simulink model "NlinCloopintcontrol"  (R2021a)
settings: Solver=VariableStepAuto  StartTime=0.0  StopTime=100  MaxStep=0.01  RelTol=1e-3
values from neighbouring files (symbols this model uses):
  g = 9.8    [Linearmodel.m]
  J = diag([2.7,3.3,5.4])    [Linearmodel.m]
  Jinv = J^-1    [Linearmodel.m]
  m = 0.254    [Linearmodel.m]
  windforce = [1;1;0]    [Linearmodel.m]
settings Model: Creator=Sirius  LastModifiedBy=Sirius

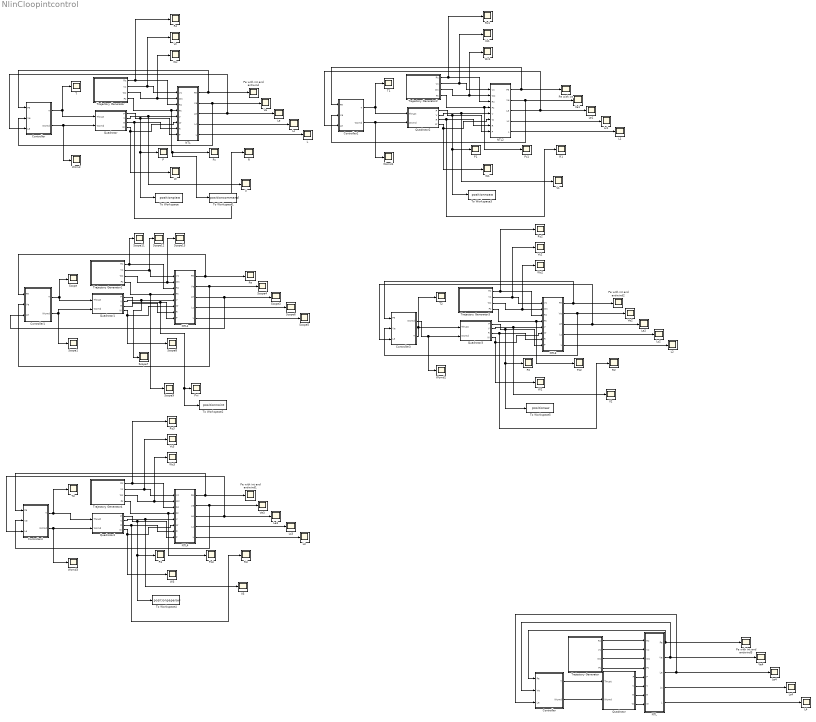
== system NlinCloopintcontrol ==
  Controller : Subsystem
  "Controller " : Subsystem
  Controller1 : MATLAB Function  TreatAsAtomicUnit=on
  Controller2 : Subsystem
  Controller3 : Subsystem
  Controller4 : Subsystem
  L{,1..4} (5 alike) : Scope
  Lc{,1..4} (5 alike) : Scope
  Le{,1..4} (5 alike) : Scope
  NTL : MATLAB Function  TreatAsAtomicUnit=on
  "NTL " : MATLAB Function  TreatAsAtomicUnit=on
  NTL1 : MATLAB Function  TreatAsAtomicUnit=on
  NTL2 : MATLAB Function  TreatAsAtomicUnit=on
  NTL3 : MATLAB Function  TreatAsAtomicUnit=on
  NTL4 : MATLAB Function  TreatAsAtomicUnit=on
  P{,1..3} (4 alike) : Scope
  Pc{,1..3} (4 alike) : Scope
  Pe : Scope
  Pe with int : Scope
  Pe with int and antiwind{,1..3} (4 alike) : Scope
  Pni : Scope
  Quadrotor : Subsystem
  "Quadrotor " : Subsystem
  Quadrotor1 : Subsystem
  Quadrotor2 : Subsystem
  Quadrotor3 : Subsystem
  Quadrotor4 : Subsystem
  R{,1..3} (4 alike) : Scope
  Rc{,1..3} (4 alike) : Scope
  Scope{,1,3..9,11..13} (12 alike) : Scope
  T{,1..3} (4 alike) : Scope
  To Workspace : ToWorkspace  VariableName=positionpiaw  SaveFormat=Timeseries  SampleTime=-1
  To Workspace1 : ToWorkspace  VariableName=positioncommand  SaveFormat=Timeseries  SampleTime=-1
  To Workspace2 : ToWorkspace  VariableName=positionnoint  SaveFormat=Timeseries  SampleTime=-1
  To Workspace3 : ToWorkspace  VariableName=positionnoaw  SaveFormat=Timeseries  SampleTime=-1
  To Workspace4 : ToWorkspace  VariableName=positionpaperaw  SaveFormat=Timeseries  SampleTime=-1
  To Workspace5 : ToWorkspace  VariableName=positionaw  SaveFormat=Timeseries  SampleTime=-1
  Trajectory Generator : Subsystem
  "Trajectory Generator " : Subsystem
  Trajectory Generator1 : Subsystem
  Trajectory Generator2 : Subsystem
  Trajectory Generator3 : Subsystem
  Trajectory Generator4 : Subsystem
  V{,1..3} (4 alike) : Scope
  Vc{,1..3} (4 alike) : Scope
  Ve{,1..4} (5 alike) : Scope
  W{,1..3} (4 alike) : Scope
  Wc{,1..3} (4 alike) : Scope
  Wcmd{,1..3} (4 alike) : Scope
  wires:
  Controller/1(T) -> Quadrotor/1(Thrust), T/1
  Trajectory Generator/3(Wc) -> Wc/1, NTL/2(Wc)
  Trajectory Generator/1(Rc) -> Rc/1, NTL/3(Rc)
  Trajectory Generator/4(Pc) -> To Workspace1/1, Pc/1, NTL/4(Pc)
  NTL/5(L) -> L/1
  NTL/4(Lc) -> Lc/1
  NTL/3(Le) -> Controller/3(Le), Le/1
  NTL/2(Ve) -> Controller/2(Ve), Ve/1
  NTL/1(Pe) -> Controller/1(Pe), Pe with int and antiwind/1
  Quadrotor/4(W) -> W/1, NTL/6(W)
  Quadrotor/1(P) -> P/1, To Workspace/1, NTL/8(P)
  Quadrotor/2(V) -> V/1, NTL/5(V)
  Quadrotor/3(R) -> R/1, NTL/7(R)
  Controller/2(Wcmd) -> Wcmd/1, Quadrotor/2(Wcmd)
  Trajectory Generator/2(Vc) -> Vc/1, NTL/1(Vc)
  Quadrotor1/4(W) -> Scope8/1, NTL1/6(W)
  Trajectory Generator1/4(Pc) -> Scope9/1, NTL1/4(Pc)
  Quadrotor1/1(P) -> To Workspace2/1, Pni/1, NTL1/8(P)
  Trajectory Generator1/1(Rc) -> Scope11/1, NTL1/3(Rc)
  Controller1/2(Wcmd) -> Quadrotor1/2(Wcmd), Scope1/1
  NTL1/1(Pe) -> Controller1/1(Pe), Pe/1
  Trajectory Generator1/3(Wc) -> Scope13/1, NTL1/2(Wc)
  Trajectory Generator1/2(Vc) -> Scope12/1, NTL1/1(Vc)
  NTL1/5(L) -> Scope5/1
  NTL1/2(Ve) -> Controller1/2(Ve), Scope4/1
  NTL1/3(Le) -> Controller1/3(Le), Scope3/1
  Controller1/1(T) -> Scope/1, Quadrotor1/1(Thrust)
  Quadrotor1/2(V) -> Scope7/1, NTL1/5(V)
  NTL1/4(Lc) -> Scope6/1
  Quadrotor1/3(R) -> NTL1/7(R)
  Quadrotor2/2(V) -> V1/1, NTL2/5(V)
  Controller2/2(Wcmd) -> Wcmd1/1, Quadrotor2/2(Wcmd)
  Controller2/1(T) -> Quadrotor2/1(Thrust), T1/1
  Trajectory Generator2/2(Vc) -> Vc1/1, NTL2/1(Vc)
  NTL2/1(Pe) -> Controller2/1(Pe), Pe with int/1
  Quadrotor2/3(R) -> R1/1, NTL2/7(R)
  Quadrotor2/1(P) -> P1/1, To Workspace3/1, NTL2/8(P)
  Trajectory Generator2/4(Pc) -> Pc1/1, NTL2/4(Pc)
  Trajectory Generator2/3(Wc) -> Wc1/1, NTL2/2(Wc)
  NTL2/4(Lc) -> Lc1/1
  NTL2/2(Ve) -> Controller2/2(Ve), Ve1/1
  NTL2/5(L) -> L1/1
  Quadrotor2/4(W) -> W1/1, NTL2/6(W)
  NTL2/3(Le) -> Controller2/3(Le), Le1/1
  Trajectory Generator2/1(Rc) -> Rc1/1, NTL2/3(Rc)
  NTL3/1(Pe) -> Controller3/1(Pe), Pe with int and antiwind2/1
  NTL3/3(Le) -> Controller3/3(Le), Le2/1
  Quadrotor3/1(P) -> P2/1, To Workspace5/1, NTL3/8(P)
  Trajectory Generator3/1(Rc) -> Rc2/1, NTL3/3(Rc)
  Quadrotor3/3(R) -> R2/1, NTL3/7(R)
  NTL3/2(Ve) -> Controller3/2(Ve), Ve2/1
  NTL3/5(L) -> L2/1
  Controller3/1(Wcmd) -> Wcmd2/1, Quadrotor3/2(Wcmd)
  Trajectory Generator3/3(Wc) -> Wc2/1, NTL3/2(Wc)
  Quadrotor3/2(V) -> V2/1, NTL3/5(V)
  Trajectory Generator3/2(Vc) -> Vc2/1, NTL3/1(Vc)
  Quadrotor3/4(W) -> W2/1, NTL3/6(W)
  NTL3/4(Lc) -> Lc2/1
  Trajectory Generator3/4(Pc) -> Pc2/1, NTL3/4(Pc)
  Controller3/2(T) -> Quadrotor3/1(Thrust), T2/1
  NTL4/1(Pe) -> Controller4/1(Pe), Pe with int and antiwind1/1
  NTL4/3(Le) -> Controller4/3(Le), Le3/1
  Quadrotor4/1(P) -> P3/1, To Workspace4/1, NTL4/8(P)
  Trajectory Generator4/1(Rc) -> Rc3/1, NTL4/3(Rc)
  Quadrotor4/3(R) -> R3/1, NTL4/7(R)
  NTL4/2(Ve) -> Controller4/2(Ve), Ve3/1
  NTL4/5(L) -> L3/1
  Trajectory Generator4/3(Wc) -> Wc3/1, NTL4/2(Wc)
  Quadrotor4/2(V) -> V3/1, NTL4/5(V)
  Trajectory Generator4/2(Vc) -> Vc3/1, NTL4/1(Vc)
  Quadrotor4/4(W) -> W3/1, NTL4/6(W)
  NTL4/4(Lc) -> Lc3/1
  Trajectory Generator4/4(Pc) -> Pc3/1, NTL4/4(Pc)
  Controller4/1(T) -> T3/1, Quadrotor4/1(Thrust)
  Controller4/2(Wcmd) -> Wcmd3/1, Quadrotor4/2(Wcmd)
  "Trajectory Generator "/1(Rc) -> "NTL "/1(Rc)
  "NTL "/5(L) -> L4/1
  "Quadrotor "/4(W) -> "NTL "/8(W)
  "Trajectory Generator "/2(Vc) -> "NTL "/2(Vc)
  "NTL "/2(Ve) -> Ve4/1, "Controller "/2(Ve)
  "Controller "/2(Wcmd) -> "Quadrotor "/2(Wcmd)
  "NTL "/1(Pe) -> Pe with int and antiwind3/1, "Controller "/1(Pe)
  "Quadrotor "/2(V) -> "NTL "/6(V)
  "NTL "/4(Lc) -> Lc4/1
  "Quadrotor "/3(R) -> "NTL "/7(R)
  "NTL "/3(Le) -> Le4/1, "Controller "/3(Le)
  "Trajectory Generator "/4(Pc) -> "NTL "/4(Pc)
  "Quadrotor "/1(P) -> "NTL "/5(P)
  "Controller "/1(T) -> "Quadrotor "/1(Thrust)
  "Trajectory Generator "/3(Wc) -> "NTL "/3(Wc)

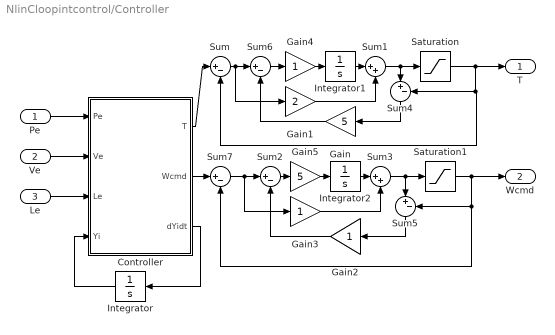
== system NlinCloopintcontrol/Controller ==
  Pe : Inport
  Ve : Inport  Port=2
  Le : Inport  Port=3
  Controller : MATLAB Function  TreatAsAtomicUnit=on
  Gain : Gain  Gain=5
  Gain1 : Gain  Gain=2
  Gain2 : Gain
  Gain3 : Gain
  Gain4 : Gain
  Gain5 : Gain  Gain=5
  Integrator : Integrator  InitialCondition=[0;0;0;0]
  Integrator1 : Integrator  InitialCondition=[0]
  Integrator2 : Integrator  InitialCondition=[0]
  Saturation : Saturate  UpperLimit=3  LowerLimit=-3
  Saturation1 : Saturate  UpperLimit=3  LowerLimit=-3
  Sum{,2,4..7} (6 alike) : Sum  Inputs=|+-
  Sum1 : Sum  Inputs=|++
  Sum3 : Sum  Inputs=|++
  T : Outport  VectorParamsAs1DForOutWhenUnconnected=off
  Wcmd : Outport  Port=2  VectorParamsAs1DForOutWhenUnconnected=off
  wires:
  Controller/3(dYidt) -> Integrator/1
  Integrator/1 -> Controller/4(Yi)
  Pe/1 -> Controller/1(Pe)
  Ve/1 -> Controller/2(Ve)
  Le/1 -> Controller/3(Le)
  Saturation/1 -> T/1, Sum/2, Sum4/2
  Controller/1(T) -> Sum/1
  Sum1/1 -> Saturation/1, Sum4/1
  Sum4/1 -> Gain/1
  Sum/1 -> Gain1/1, Sum6/1
  Gain4/1 -> Integrator1/1
  Sum2/1 -> Gain5/1
  Gain2/1 -> Sum2/2
  Sum3/1 -> Sum5/1, Saturation1/1
  Saturation1/1 -> Wcmd/1, Sum7/2, Sum5/2
  Gain5/1 -> Integrator2/1
  Sum5/1 -> Gain2/1
  Controller/2(Wcmd) -> Sum7/1
  Sum6/1 -> Gain4/1
  Gain/1 -> Sum6/2
  Sum7/1 -> Gain3/1, Sum2/1
  Integrator1/1 -> Sum1/1
  Gain1/1 -> Sum1/2
  Integrator2/1 -> Sum3/1
  Gain3/1 -> Sum3/2

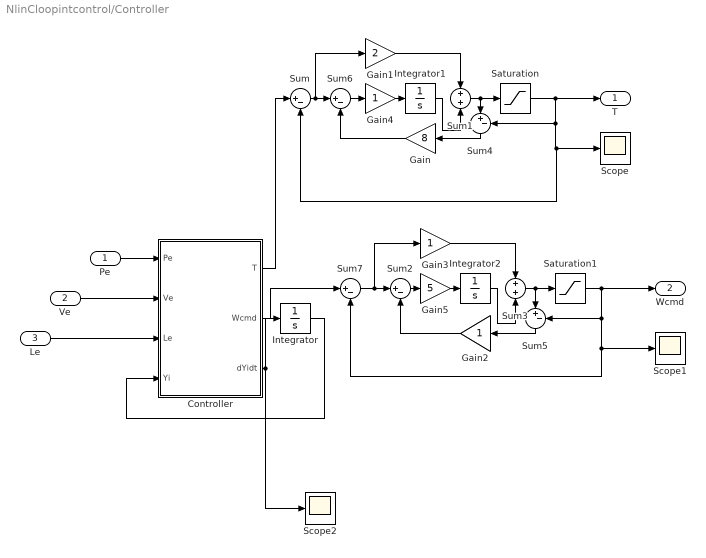
== system NlinCloopintcontrol/Controller  ==
  Pe : Inport
  Ve : Inport  Port=2
  Le : Inport  Port=3
  Controller : MATLAB Function  TreatAsAtomicUnit=on
  Gain : Gain  Gain=8
  Gain1 : Gain  Gain=2
  Gain2 : Gain
  Gain3 : Gain
  Gain4 : Gain
  Gain5 : Gain  Gain=5
  Integrator : Integrator  InitialCondition=[0;0;0;0]
  Integrator1 : Integrator  InitialCondition=[0]
  Integrator2 : Integrator  InitialCondition=[0]
  Saturation : Saturate  UpperLimit=3  LowerLimit=-3
  Saturation1 : Saturate  UpperLimit=3  LowerLimit=-3
  Scope : Scope
  Scope1 : Scope
  Scope2 : Scope
  Sum{,2,4..7} (6 alike) : Sum  Inputs=|+-
  Sum1 : Sum
  Sum3 : Sum
  T : Outport  VectorParamsAs1DForOutWhenUnconnected=off
  Wcmd : Outport  Port=2  VectorParamsAs1DForOutWhenUnconnected=off
  wires:
  Controller/3(dYidt) -> Integrator/1, Scope2/1
  Integrator/1 -> Controller/4(Yi)
  Pe/1 -> Controller/1(Pe)
  Ve/1 -> Controller/2(Ve)
  Le/1 -> Controller/3(Le)
  Saturation/1 -> T/1, Sum/2, Scope/1, Sum4/2
  Controller/1(T) -> Sum/1
  Gain1/1 -> Sum1/1
  Sum1/1 -> Saturation/1, Sum4/1
  Integrator1/1 -> Sum1/2
  Sum4/1 -> Gain/1
  Sum/1 -> Gain1/1, Sum6/1
  Gain4/1 -> Integrator1/1
  Sum2/1 -> Gain5/1
  Gain3/1 -> Sum3/1
  Gain2/1 -> Sum2/2
  Sum3/1 -> Sum5/1, Saturation1/1
  Integrator2/1 -> Sum3/2
  Saturation1/1 -> Wcmd/1, Sum7/2, Scope1/1, Sum5/2
  Gain5/1 -> Integrator2/1
  Sum5/1 -> Gain2/1
  Controller/2(Wcmd) -> Sum7/1
  Sum6/1 -> Gain4/1
  Gain/1 -> Sum6/2
  Sum7/1 -> Gain3/1, Sum2/1

== system NlinCloopintcontrol/Controller2 ==
  Pe : Inport
  Ve : Inport  Port=2
  Le : Inport  Port=3
  Controller : MATLAB Function  TreatAsAtomicUnit=on
  Integrator : Integrator  InitialCondition=[0;0;0;0]
  Scope : Scope
  Scope1 : Scope
  To Workspace : ToWorkspace  VariableName=xnoaw  SaveFormat=Timeseries  SampleTime=-1
  To Workspace1 : ToWorkspace  VariableName=unoaw  SaveFormat=Timeseries  SampleTime=-1
  T : Outport  VectorParamsAs1DForOutWhenUnconnected=off
  Wcmd : Outport  Port=2  VectorParamsAs1DForOutWhenUnconnected=off
  wires:
  Controller/3(dYidt) -> Integrator/1
  Integrator/1 -> Controller/4(Yi)
  Pe/1 -> Controller/1(Pe)
  Ve/1 -> Controller/2(Ve)
  Le/1 -> Controller/3(Le)
  Controller/4(x) -> To Workspace/1
  Controller/5(u) -> To Workspace1/1
  Controller/1(T) -> Scope/1, T/1
  Controller/2(Wcmd) -> Scope1/1, Wcmd/1

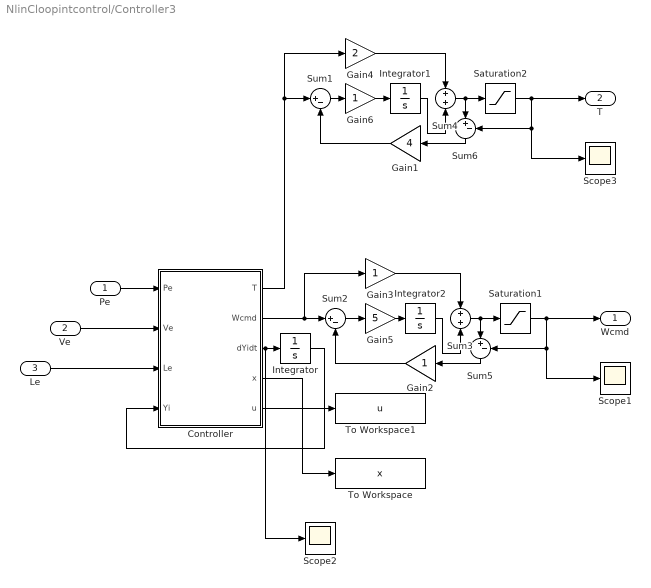
== system NlinCloopintcontrol/Controller3 ==
  Pe : Inport
  Ve : Inport  Port=2
  Le : Inport  Port=3
  Controller : MATLAB Function  TreatAsAtomicUnit=on
  Gain1 : Gain  Gain=4
  Gain2 : Gain
  Gain3 : Gain
  Gain4 : Gain  Gain=2
  Gain5 : Gain  Gain=5
  Gain6 : Gain
  Integrator : Integrator  InitialCondition=[0;0;0;0]
  Integrator1 : Integrator  InitialCondition=[0]
  Integrator2 : Integrator  InitialCondition=[0]
  Saturation1 : Saturate  UpperLimit=3  LowerLimit=-3
  Saturation2 : Saturate  UpperLimit=3  LowerLimit=-3
  Scope1 : Scope
  Scope2 : Scope
  Scope3 : Scope
  Sum{1..2,5..6} (4 alike) : Sum  Inputs=|+-
  Sum3 : Sum
  Sum4 : Sum
  To Workspace : ToWorkspace  VariableName=x  SaveFormat=Timeseries  SampleTime=-1
  To Workspace1 : ToWorkspace  VariableName=u  SaveFormat=Timeseries  SampleTime=-1
  Wcmd : Outport  VectorParamsAs1DForOutWhenUnconnected=off
  T : Outport  Port=2  VectorParamsAs1DForOutWhenUnconnected=off
  wires:
  Controller/3(dYidt) -> Scope2/1, Integrator/1
  Integrator/1 -> Controller/4(Yi)
  Pe/1 -> Controller/1(Pe)
  Ve/1 -> Controller/2(Ve)
  Le/1 -> Controller/3(Le)
  Controller/4(x) -> To Workspace/1
  Controller/5(u) -> To Workspace1/1
  Controller/1(T) -> Gain4/1, Sum1/1
  Sum2/1 -> Gain5/1
  Gain3/1 -> Sum3/1
  Gain2/1 -> Sum2/2
  Sum3/1 -> Sum5/1, Saturation1/1
  Integrator2/1 -> Sum3/2
  Saturation1/1 -> Wcmd/1, Scope1/1, Sum5/2
  Gain5/1 -> Integrator2/1
  Sum5/1 -> Gain2/1
  Controller/2(Wcmd) -> Gain3/1, Sum2/1
  Integrator1/1 -> Sum4/2
  Gain1/1 -> Sum1/2
  Gain4/1 -> Sum4/1
  Sum4/1 -> Sum6/1, Saturation2/1
  Saturation2/1 -> T/1, Scope3/1, Sum6/2
  Gain6/1 -> Integrator1/1
  Sum6/1 -> Gain1/1
  Sum1/1 -> Gain6/1

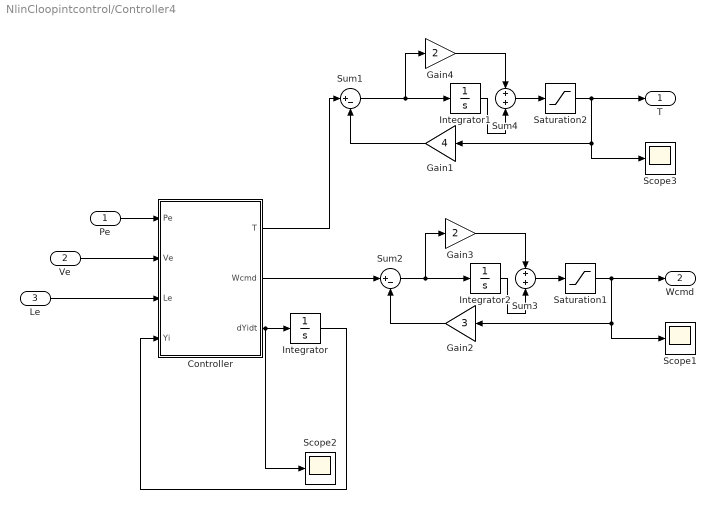
== system NlinCloopintcontrol/Controller4 ==
  Pe : Inport
  Ve : Inport  Port=2
  Le : Inport  Port=3
  Controller : MATLAB Function  TreatAsAtomicUnit=on
  Gain1 : Gain  Gain=4
  Gain2 : Gain  Gain=3
  Gain3 : Gain  Gain=2
  Gain4 : Gain  Gain=2
  Integrator : Integrator  InitialCondition=[0;0;0;0]
  Integrator1 : Integrator  InitialCondition=[0]
  Integrator2 : Integrator  InitialCondition=[0]
  Saturation1 : Saturate  UpperLimit=3  LowerLimit=-3
  Saturation2 : Saturate  UpperLimit=3  LowerLimit=-3
  Scope1 : Scope
  Scope2 : Scope
  Scope3 : Scope
  Sum1 : Sum  Inputs=|+-
  Sum2 : Sum  Inputs=|+-
  Sum3 : Sum
  Sum4 : Sum
  T : Outport  VectorParamsAs1DForOutWhenUnconnected=off
  Wcmd : Outport  Port=2  VectorParamsAs1DForOutWhenUnconnected=off
  wires:
  Controller/3(dYidt) -> Scope2/1, Integrator/1
  Pe/1 -> Controller/1(Pe)
  Ve/1 -> Controller/2(Ve)
  Le/1 -> Controller/3(Le)
  Controller/1(T) -> Sum1/1
  Controller/2(Wcmd) -> Sum2/1
  Sum4/1 -> Saturation2/1
  Integrator1/1 -> Sum4/2
  Gain4/1 -> Sum4/1
  Saturation2/1 -> T/1, Gain1/1, Scope3/1
  Sum1/1 -> Gain4/1, Integrator1/1
  Gain1/1 -> Sum1/2
  Integrator/1 -> Controller/4(Yi)
  Sum3/1 -> Saturation1/1
  Integrator2/1 -> Sum3/2
  Gain3/1 -> Sum3/1
  Saturation1/1 -> Wcmd/1, Gain2/1, Scope1/1
  Sum2/1 -> Gain3/1, Integrator2/1
  Gain2/1 -> Sum2/2

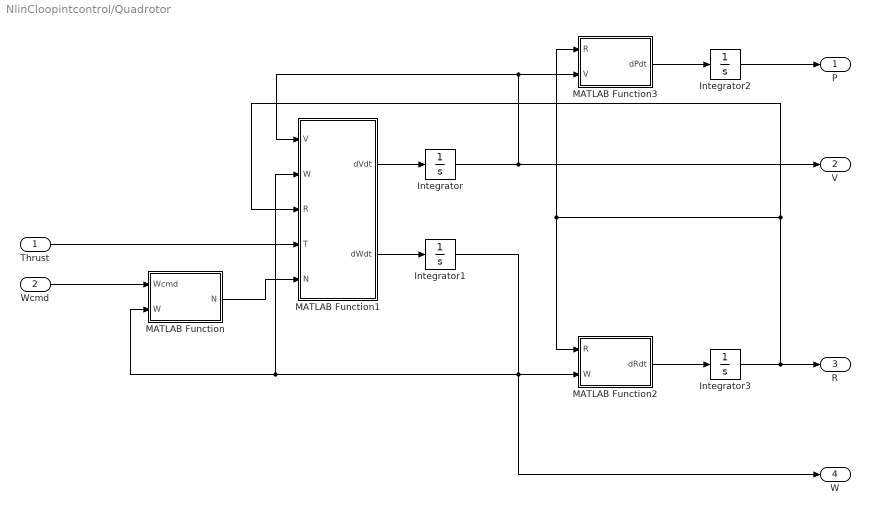
== system NlinCloopintcontrol/Quadrotor ==
  Thrust : Inport
  Wcmd : Inport  Port=2
  Integrator : Integrator  InitialCondition=[0;0;0]
  Integrator1 : Integrator  InitialCondition=[0;0;0]
  Integrator2 : Integrator  InitialCondition=[0;1;0]
  Integrator3 : Integrator  InitialCondition=eye(3)
  MATLAB Function : MATLAB Function  TreatAsAtomicUnit=on
  MATLAB Function1 : MATLAB Function  TreatAsAtomicUnit=on
  MATLAB Function2 : MATLAB Function  TreatAsAtomicUnit=on
  MATLAB Function3 : MATLAB Function  TreatAsAtomicUnit=on
  P : Outport
  V : Outport  Port=2
  R : Outport  Port=3
  W : Outport  Port=4
  wires:
  MATLAB Function2/1(dRdt) -> Integrator3/1
  Wcmd/1 -> MATLAB Function/1(Wcmd)
  MATLAB Function1/1(dVdt) -> Integrator/1
  Thrust/1 -> MATLAB Function1/4(T)
  MATLAB Function1/2(dWdt) -> Integrator1/1
  MATLAB Function/1(N) -> MATLAB Function1/5(N)
  MATLAB Function3/1(dPdt) -> Integrator2/1
  Integrator/1 -> V/1, MATLAB Function1/1(V), MATLAB Function3/2(V)
  Integrator3/1 -> MATLAB Function1/3(R), MATLAB Function3/1(R), MATLAB Function2/1(R), R/1
  Integrator1/1 -> MATLAB Function1/2(W), MATLAB Function/2(W), W/1, MATLAB Function2/2(W)
  Integrator2/1 -> P/1

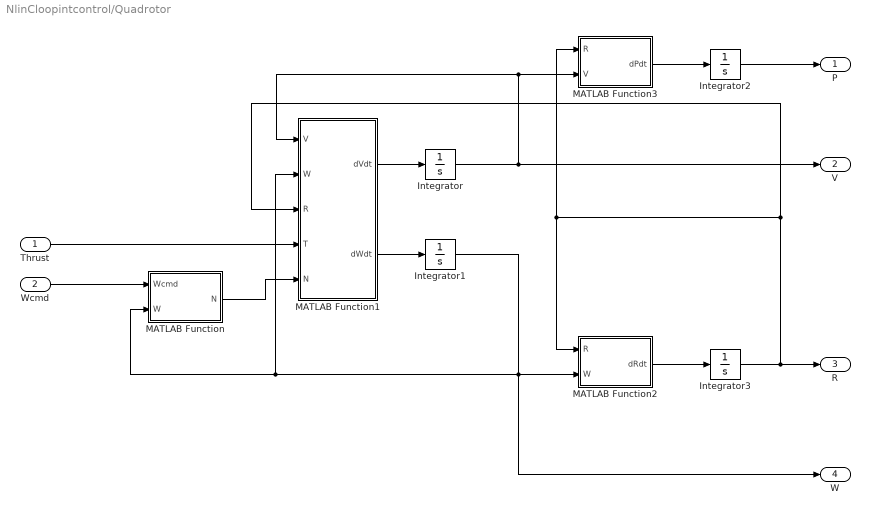
== system NlinCloopintcontrol/Quadrotor  ==
  Thrust : Inport
  Wcmd : Inport  Port=2
  Integrator : Integrator  InitialCondition=[0;0;0]
  Integrator1 : Integrator  InitialCondition=[0;0;0]
  Integrator2 : Integrator  InitialCondition=[0;1;0]
  Integrator3 : Integrator  InitialCondition=eye(3)
  MATLAB Function : MATLAB Function  TreatAsAtomicUnit=on
  MATLAB Function1 : MATLAB Function  TreatAsAtomicUnit=on
  MATLAB Function2 : MATLAB Function  TreatAsAtomicUnit=on
  MATLAB Function3 : MATLAB Function  TreatAsAtomicUnit=on
  P : Outport
  V : Outport  Port=2
  R : Outport  Port=3
  W : Outport  Port=4
  wires:
  MATLAB Function2/1(dRdt) -> Integrator3/1
  Wcmd/1 -> MATLAB Function/1(Wcmd)
  MATLAB Function1/1(dVdt) -> Integrator/1
  Thrust/1 -> MATLAB Function1/4(T)
  MATLAB Function1/2(dWdt) -> Integrator1/1
  MATLAB Function/1(N) -> MATLAB Function1/5(N)
  MATLAB Function3/1(dPdt) -> Integrator2/1
  Integrator/1 -> V/1, MATLAB Function1/1(V), MATLAB Function3/2(V)
  Integrator3/1 -> MATLAB Function1/3(R), MATLAB Function3/1(R), MATLAB Function2/1(R), R/1
  Integrator1/1 -> MATLAB Function1/2(W), MATLAB Function/2(W), W/1, MATLAB Function2/2(W)
  Integrator2/1 -> P/1

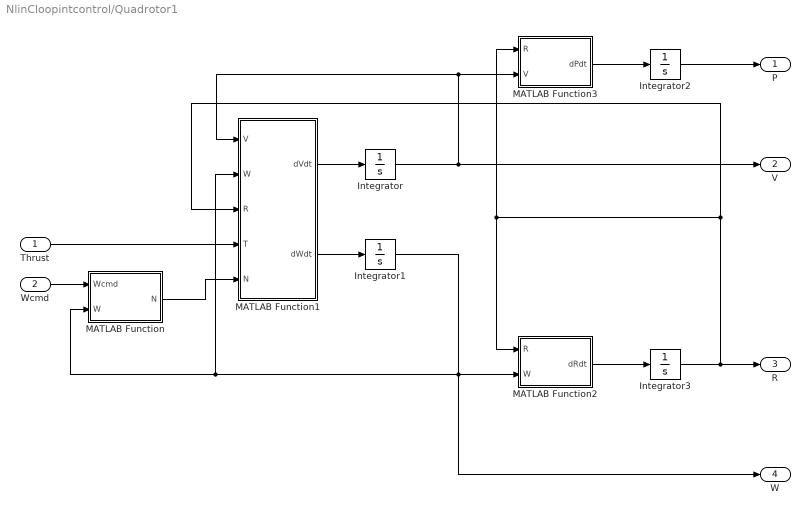
== system NlinCloopintcontrol/Quadrotor1 ==
  Thrust : Inport
  Wcmd : Inport  Port=2
  Integrator : Integrator  InitialCondition=[0;0;0]
  Integrator1 : Integrator  InitialCondition=[0;0;0]
  Integrator2 : Integrator  InitialCondition=[0;1;0]
  Integrator3 : Integrator  InitialCondition=eye(3)
  MATLAB Function : MATLAB Function  TreatAsAtomicUnit=on
  MATLAB Function1 : MATLAB Function  TreatAsAtomicUnit=on
  MATLAB Function2 : MATLAB Function  TreatAsAtomicUnit=on
  MATLAB Function3 : MATLAB Function  TreatAsAtomicUnit=on
  P : Outport
  V : Outport  Port=2
  R : Outport  Port=3
  W : Outport  Port=4
  wires:
  MATLAB Function2/1(dRdt) -> Integrator3/1
  Wcmd/1 -> MATLAB Function/1(Wcmd)
  MATLAB Function1/1(dVdt) -> Integrator/1
  Thrust/1 -> MATLAB Function1/4(T)
  MATLAB Function1/2(dWdt) -> Integrator1/1
  MATLAB Function/1(N) -> MATLAB Function1/5(N)
  MATLAB Function3/1(dPdt) -> Integrator2/1
  Integrator/1 -> V/1, MATLAB Function1/1(V), MATLAB Function3/2(V)
  Integrator3/1 -> MATLAB Function1/3(R), MATLAB Function3/1(R), MATLAB Function2/1(R), R/1
  Integrator1/1 -> MATLAB Function1/2(W), MATLAB Function/2(W), W/1, MATLAB Function2/2(W)
  Integrator2/1 -> P/1

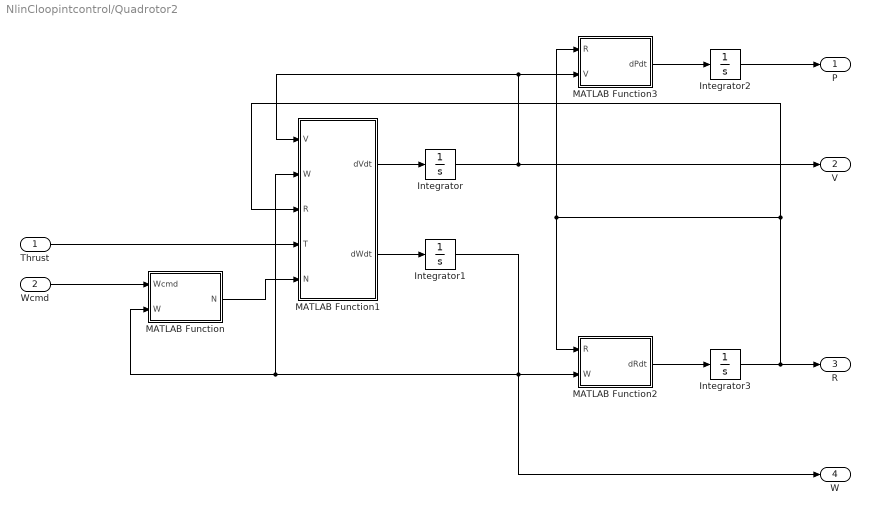
== system NlinCloopintcontrol/Quadrotor2 ==
  Thrust : Inport
  Wcmd : Inport  Port=2
  Integrator : Integrator  InitialCondition=[0;0;0]
  Integrator1 : Integrator  InitialCondition=[0;0;0]
  Integrator2 : Integrator  InitialCondition=[0;1;0]
  Integrator3 : Integrator  InitialCondition=eye(3)
  MATLAB Function : MATLAB Function  TreatAsAtomicUnit=on
  MATLAB Function1 : MATLAB Function  TreatAsAtomicUnit=on
  MATLAB Function2 : MATLAB Function  TreatAsAtomicUnit=on
  MATLAB Function3 : MATLAB Function  TreatAsAtomicUnit=on
  P : Outport
  V : Outport  Port=2
  R : Outport  Port=3
  W : Outport  Port=4
  wires:
  MATLAB Function2/1(dRdt) -> Integrator3/1
  Wcmd/1 -> MATLAB Function/1(Wcmd)
  MATLAB Function1/1(dVdt) -> Integrator/1
  Thrust/1 -> MATLAB Function1/4(T)
  MATLAB Function1/2(dWdt) -> Integrator1/1
  MATLAB Function/1(N) -> MATLAB Function1/5(N)
  MATLAB Function3/1(dPdt) -> Integrator2/1
  Integrator/1 -> V/1, MATLAB Function1/1(V), MATLAB Function3/2(V)
  Integrator3/1 -> MATLAB Function1/3(R), MATLAB Function3/1(R), MATLAB Function2/1(R), R/1
  Integrator1/1 -> MATLAB Function1/2(W), MATLAB Function/2(W), W/1, MATLAB Function2/2(W)
  Integrator2/1 -> P/1

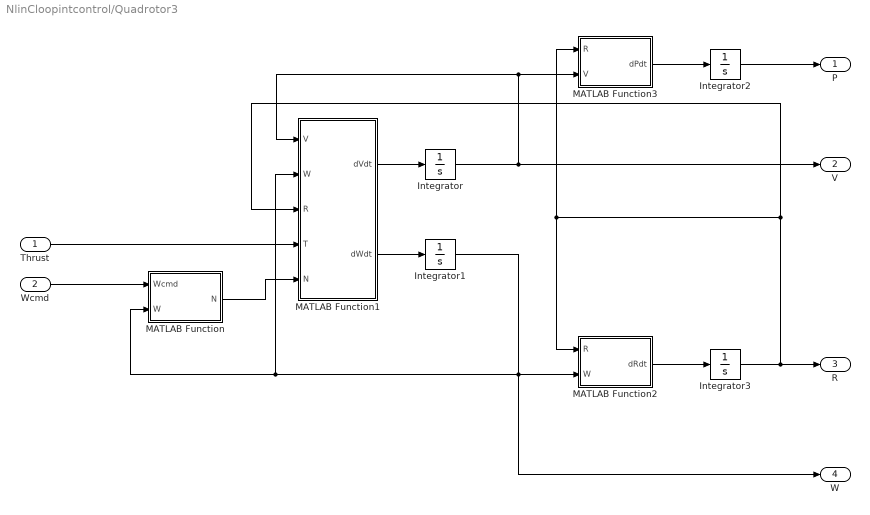
== system NlinCloopintcontrol/Quadrotor3 ==
  Thrust : Inport
  Wcmd : Inport  Port=2
  Integrator : Integrator  InitialCondition=[0;0;0]
  Integrator1 : Integrator  InitialCondition=[0;0;0]
  Integrator2 : Integrator  InitialCondition=[0;1;0]
  Integrator3 : Integrator  InitialCondition=eye(3)
  MATLAB Function : MATLAB Function  TreatAsAtomicUnit=on
  MATLAB Function1 : MATLAB Function  TreatAsAtomicUnit=on
  MATLAB Function2 : MATLAB Function  TreatAsAtomicUnit=on
  MATLAB Function3 : MATLAB Function  TreatAsAtomicUnit=on
  P : Outport
  V : Outport  Port=2
  R : Outport  Port=3
  W : Outport  Port=4
  wires:
  MATLAB Function2/1(dRdt) -> Integrator3/1
  Wcmd/1 -> MATLAB Function/1(Wcmd)
  MATLAB Function1/1(dVdt) -> Integrator/1
  Thrust/1 -> MATLAB Function1/4(T)
  MATLAB Function1/2(dWdt) -> Integrator1/1
  MATLAB Function/1(N) -> MATLAB Function1/5(N)
  MATLAB Function3/1(dPdt) -> Integrator2/1
  Integrator/1 -> V/1, MATLAB Function1/1(V), MATLAB Function3/2(V)
  Integrator3/1 -> MATLAB Function1/3(R), MATLAB Function3/1(R), MATLAB Function2/1(R), R/1
  Integrator1/1 -> MATLAB Function1/2(W), MATLAB Function/2(W), W/1, MATLAB Function2/2(W)
  Integrator2/1 -> P/1

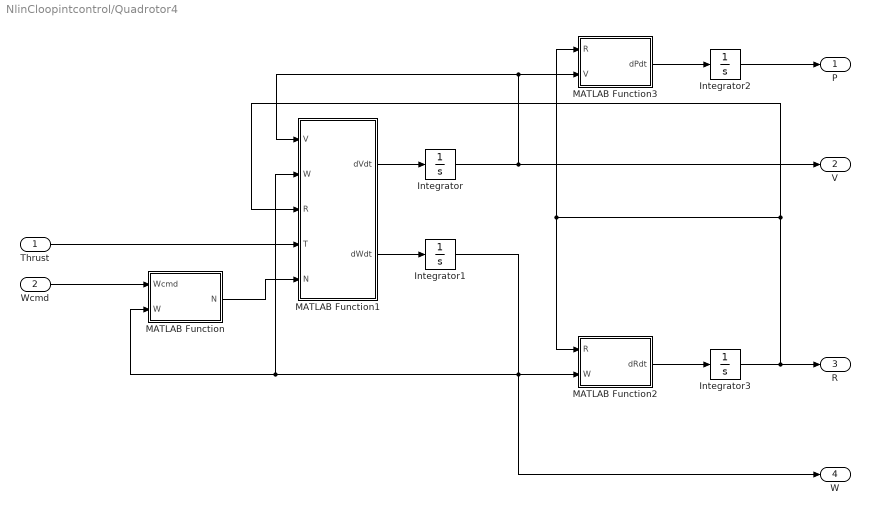
== system NlinCloopintcontrol/Quadrotor4 ==
  Thrust : Inport
  Wcmd : Inport  Port=2
  Integrator : Integrator  InitialCondition=[0;0;0]
  Integrator1 : Integrator  InitialCondition=[0;0;0]
  Integrator2 : Integrator  InitialCondition=[0;1;0]
  Integrator3 : Integrator  InitialCondition=eye(3)
  MATLAB Function : MATLAB Function  TreatAsAtomicUnit=on
  MATLAB Function1 : MATLAB Function  TreatAsAtomicUnit=on
  MATLAB Function2 : MATLAB Function  TreatAsAtomicUnit=on
  MATLAB Function3 : MATLAB Function  TreatAsAtomicUnit=on
  P : Outport
  V : Outport  Port=2
  R : Outport  Port=3
  W : Outport  Port=4
  wires:
  MATLAB Function2/1(dRdt) -> Integrator3/1
  Wcmd/1 -> MATLAB Function/1(Wcmd)
  MATLAB Function1/1(dVdt) -> Integrator/1
  Thrust/1 -> MATLAB Function1/4(T)
  MATLAB Function1/2(dWdt) -> Integrator1/1
  MATLAB Function/1(N) -> MATLAB Function1/5(N)
  MATLAB Function3/1(dPdt) -> Integrator2/1
  Integrator/1 -> V/1, MATLAB Function1/1(V), MATLAB Function3/2(V)
  Integrator3/1 -> MATLAB Function1/3(R), MATLAB Function3/1(R), MATLAB Function2/1(R), R/1
  Integrator1/1 -> MATLAB Function1/2(W), MATLAB Function/2(W), W/1, MATLAB Function2/2(W)
  Integrator2/1 -> P/1

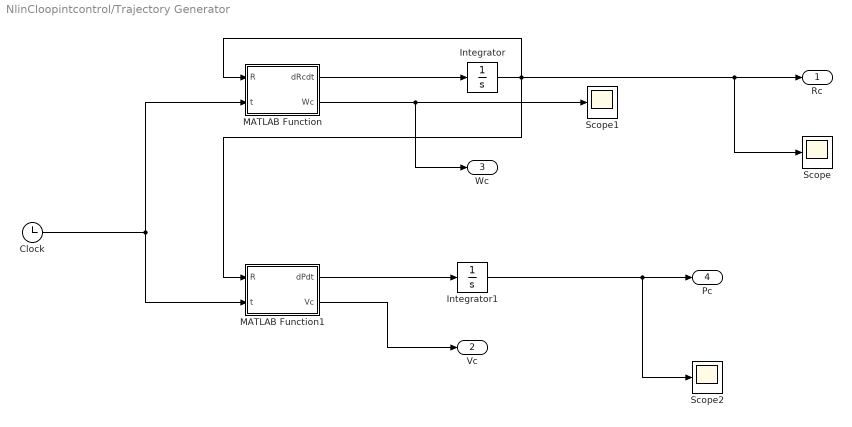
== system NlinCloopintcontrol/Trajectory Generator ==
  Clock : Clock
  Integrator : Integrator  InitialCondition=eye(3)
  Integrator1 : Integrator  InitialCondition=[0;0;0]
  MATLAB Function : MATLAB Function  TreatAsAtomicUnit=on
  MATLAB Function1 : MATLAB Function  TreatAsAtomicUnit=on
  Scope : Scope
  Scope1 : Scope
  Scope2 : Scope
  Rc : Outport
  Vc : Outport  Port=2
  Wc : Outport  Port=3
  Pc : Outport  Port=4
  wires:
  MATLAB Function1/1(dPdt) -> Integrator1/1
  Integrator1/1 -> Scope2/1, Pc/1
  Integrator/1 -> MATLAB Function1/1(R), MATLAB Function/1(R), Scope/1, Rc/1
  MATLAB Function/2(Wc) -> Wc/1, Scope1/1
  MATLAB Function1/2(Vc) -> Vc/1
  Clock/1 -> MATLAB Function/2(t), MATLAB Function1/2(t)
  MATLAB Function/1(dRcdt) -> Integrator/1

== system NlinCloopintcontrol/Trajectory Generator  ==
  Clock : Clock
  Integrator : Integrator  InitialCondition=eye(3)
  Integrator1 : Integrator  InitialCondition=[0;0;0]
  MATLAB Function : MATLAB Function  TreatAsAtomicUnit=on
  MATLAB Function1 : MATLAB Function  TreatAsAtomicUnit=on
  Scope : Scope
  Scope1 : Scope
  Scope2 : Scope
  Rc : Outport
  Vc : Outport  Port=2
  Wc : Outport  Port=3
  Pc : Outport  Port=4
  wires:
  MATLAB Function1/1(dPdt) -> Integrator1/1
  Integrator1/1 -> Scope2/1, Pc/1
  Integrator/1 -> MATLAB Function1/1(R), MATLAB Function/1(R), Scope/1, Rc/1
  MATLAB Function/2(Wc) -> Wc/1, Scope1/1
  MATLAB Function1/2(Vc) -> Vc/1
  Clock/1 -> MATLAB Function/2(t), MATLAB Function1/2(t)
  MATLAB Function/1(dRcdt) -> Integrator/1

== system NlinCloopintcontrol/Trajectory Generator1 ==
  Clock : Clock
  Integrator : Integrator  InitialCondition=eye(3)
  Integrator1 : Integrator  InitialCondition=[0;0;0]
  MATLAB Function : MATLAB Function  TreatAsAtomicUnit=on
  MATLAB Function1 : MATLAB Function  TreatAsAtomicUnit=on
  Scope : Scope
  Scope1 : Scope
  Scope2 : Scope
  Rc : Outport
  Vc : Outport  Port=2
  Wc : Outport  Port=3
  Pc : Outport  Port=4
  wires:
  MATLAB Function1/1(dPdt) -> Integrator1/1
  Integrator1/1 -> Scope2/1, Pc/1
  Integrator/1 -> MATLAB Function1/1(R), MATLAB Function/1(R), Scope/1, Rc/1
  MATLAB Function/2(Wc) -> Wc/1, Scope1/1
  MATLAB Function1/2(Vc) -> Vc/1
  Clock/1 -> MATLAB Function/2(t), MATLAB Function1/2(t)
  MATLAB Function/1(dRcdt) -> Integrator/1

== system NlinCloopintcontrol/Trajectory Generator2 ==
  Clock : Clock
  Integrator : Integrator  InitialCondition=eye(3)
  Integrator1 : Integrator  InitialCondition=[0;0;0]
  MATLAB Function : MATLAB Function  TreatAsAtomicUnit=on
  MATLAB Function1 : MATLAB Function  TreatAsAtomicUnit=on
  Scope : Scope
  Scope1 : Scope
  Scope2 : Scope
  Rc : Outport
  Vc : Outport  Port=2
  Wc : Outport  Port=3
  Pc : Outport  Port=4
  wires:
  MATLAB Function1/1(dPdt) -> Integrator1/1
  Integrator1/1 -> Scope2/1, Pc/1
  Integrator/1 -> MATLAB Function1/1(R), MATLAB Function/1(R), Scope/1, Rc/1
  MATLAB Function/2(Wc) -> Wc/1, Scope1/1
  MATLAB Function1/2(Vc) -> Vc/1
  Clock/1 -> MATLAB Function/2(t), MATLAB Function1/2(t)
  MATLAB Function/1(dRcdt) -> Integrator/1

== system NlinCloopintcontrol/Trajectory Generator3 ==
  Clock : Clock
  Integrator : Integrator  InitialCondition=eye(3)
  Integrator1 : Integrator  InitialCondition=[0;0;0]
  MATLAB Function : MATLAB Function  TreatAsAtomicUnit=on
  MATLAB Function1 : MATLAB Function  TreatAsAtomicUnit=on
  Scope : Scope
  Scope1 : Scope
  Scope2 : Scope
  Rc : Outport
  Vc : Outport  Port=2
  Wc : Outport  Port=3
  Pc : Outport  Port=4
  wires:
  MATLAB Function1/1(dPdt) -> Integrator1/1
  Integrator1/1 -> Scope2/1, Pc/1
  Integrator/1 -> MATLAB Function1/1(R), MATLAB Function/1(R), Scope/1, Rc/1
  MATLAB Function/2(Wc) -> Wc/1, Scope1/1
  MATLAB Function1/2(Vc) -> Vc/1
  Clock/1 -> MATLAB Function/2(t), MATLAB Function1/2(t)
  MATLAB Function/1(dRcdt) -> Integrator/1

== system NlinCloopintcontrol/Trajectory Generator4 ==
  Clock : Clock
  Integrator : Integrator  InitialCondition=eye(3)
  Integrator1 : Integrator  InitialCondition=[0;0;0]
  MATLAB Function : MATLAB Function  TreatAsAtomicUnit=on
  MATLAB Function1 : MATLAB Function  TreatAsAtomicUnit=on
  Scope : Scope
  Scope1 : Scope
  Scope2 : Scope
  Rc : Outport
  Vc : Outport  Port=2
  Wc : Outport  Port=3
  Pc : Outport  Port=4
  wires:
  MATLAB Function1/1(dPdt) -> Integrator1/1
  Integrator1/1 -> Scope2/1, Pc/1
  Integrator/1 -> MATLAB Function1/1(R), MATLAB Function/1(R), Scope/1, Rc/1
  MATLAB Function/2(Wc) -> Wc/1, Scope1/1
  MATLAB Function1/2(Vc) -> Vc/1
  Clock/1 -> MATLAB Function/2(t), MATLAB Function1/2(t)
  MATLAB Function/1(dRcdt) -> Integrator/1

== matlab function NlinCloopintcontrol/Controller2/Controller ==
  data: Pe input; T output; Ve input; Le input; Wcmd output; Ki parameter; Yi input; dYidt output; x output; u output
function [T,Wcmd,dYidt,x,u]=Controller(Pe,Ve,Le,Ki,Yi)
x=[Pe;Ve;Le;Yi];
u=-Ki*x;
T=u(1);
Wcmd=u(2:4);
dYidt=[Pe;Le(3)];
end

== matlab function NlinCloopintcontrol/NTL1 ==
  data: Vc input; Pe output; Wc input; Rc input; Pc input; V input; W input; R input; P input; Ve output; Le output; Lc output; L output
function [Pe,Ve,Le,Lc,L] = NLT(Vc,Wc,Rc,Pc,V,W,R,P)
Rc2b=R'*Rc;
Ve=V-Vc;
Pe=R'*(P-Pc);
Re=Rc'*R;
L=Rmat2PRY(R)*180/pi;
Lc=Rmat2PRY(Rc)*180/pi;
Le=Rmat2PRY(Re);
end

== matlab function NlinCloopintcontrol/Quadrotor1/MATLAB Function ==
  data: Wcmd input; N output; W input
function N = Wcontorl(Wcmd,W)
N=1000*(Wcmd-W);
end

== matlab function NlinCloopintcontrol/Quadrotor1/MATLAB Function1 ==
  data: V input; dVdt output; W input; R input; T input; N input; dWdt output; Jinv parameter; m parameter; g parameter; J parameter; windforce parameter
function [dVdt,dWdt]=QDyanamics(V,W,R,T,N,Jinv, m, g, J, windforce)
dVdt=-Skew(W)*V+1/m*([0;0;-T]+R'*[0;0;m*g]+ windforce);
dWdt=-Jinv*Skew(W)*J*W+Jinv*N;
end

== matlab function NlinCloopintcontrol/Quadrotor1/MATLAB Function2 ==
  data: R input; dRdt output; W input
function dRdt=dRdt(R,W)
dRdt=R*Skew(W);
end

== matlab function NlinCloopintcontrol/Quadrotor1/MATLAB Function3 ==
  data: R input; dPdt output; V input
function dPdt=dPdt(R,V)
dPdt=R*V;
end

== matlab function NlinCloopintcontrol/Trajectory Generator1/MATLAB Function ==
  data: R input; dRcdt output; t input; Wc output
function [dRcdt,Wc] =dRdt(R,t)

Wc=[0;0;0];
if((t>=19.5)&&(t<=20.5))
    Wc=[0;0;pi/2];
end
if((t>=39.5)&&(t<=40.5))
    Wc=[0;0;pi/2];
end
if((t>=59.5)&&(t<=60.5))
    Wc=[0;0;pi/2];
end
dRcdt=R*Skew(Wc);
end

== matlab function NlinCloopintcontrol/Trajectory Generator/MATLAB Function ==
  data: R input; dRcdt output; t input; Wc output
function [dRcdt,Wc] =dRdt(R,t)

Wc=[0;0;0];
if((t>=19.5)&&(t<=20.5))
    Wc=[0;0;pi/2];
end
if((t>=39.5)&&(t<=40.5))
    Wc=[0;0;pi/2];
end
if((t>=59.5)&&(t<=60.5))
    Wc=[0;0;pi/2];
end
dRcdt=R*Skew(Wc);
end

== matlab function NlinCloopintcontrol/Trajectory Generator1/MATLAB Function1 ==
  data: R input; dPdt output; t input; Vc output
function [dPdt,Vc] = dPdt(R,t)
Vc=[0.5;0;0];
dPdt=R*Vc;
end

== matlab function NlinCloopintcontrol/NTL2 ==
  data: Vc input; Pe output; Wc input; Rc input; Pc input; V input; W input; R input; P input; Ve output; Le output; Lc output; L output
function [Pe,Ve,Le,Lc,L] = NLT(Vc,Wc,Rc,Pc,V,W,R,P)
Rc2b=R'*Rc;
Ve=V-Vc;
Re=Rc'*R;
%Pe=R'*(P-Pc);
Pe=R'*(P-Pc);
L=Rmat2PRY(R)*180/pi;
Lc=Rmat2PRY(Rc)*180/pi;
Le=Rmat2PRY(Re);
end

== matlab function NlinCloopintcontrol/Controller/Controller ==
  data: Pe input; T output; Ve input; Le input; Wcmd output; Ki parameter; Yi input; dYidt output
function [T,Wcmd,dYidt]=Controller(Pe,Ve,Le,Ki,Yi)
x=[Pe;Ve;Le;Yi];
u=-Ki*x;
T=u(1);
Wcmd=u(2:4);
dYidt=[Pe;Le(3)];
end

== matlab function NlinCloopintcontrol/Quadrotor2/MATLAB Function ==
  data: Wcmd input; N output; W input
function N = Wcontorl(Wcmd,W)
N=1000*(Wcmd-W);
end

== matlab function NlinCloopintcontrol/Quadrotor2/MATLAB Function1 ==
  data: V input; dVdt output; W input; R input; T input; N input; dWdt output; Jinv parameter; m parameter; g parameter; J parameter; windforce parameter
function [dVdt,dWdt]=QDyanamics(V,W,R,T,N,Jinv, m, g, J, windforce)
dVdt=-Skew(W)*V+1/m*([0;0;-T]+R'*[0;0;m*g]+windforce);
dWdt=-Jinv*Skew(W)*J*W+Jinv*N;
end

== matlab function NlinCloopintcontrol/Quadrotor2/MATLAB Function2 ==
  data: R input; dRdt output; W input
function dRdt=dRdt(R,W)
dRdt=R*Skew(W);
end

== matlab function NlinCloopintcontrol/Quadrotor2/MATLAB Function3 ==
  data: R input; dPdt output; V input
function dPdt=dPdt(R,V)
dPdt=R*V;
end

== matlab function NlinCloopintcontrol/Trajectory Generator2/MATLAB Function ==
  data: R input; dRcdt output; t input; Wc output
function [dRcdt,Wc] =dRdt(R,t)

Wc=[0;0;0];
if((t>=19.5)&&(t<=20.5))
    Wc=[0;0;pi/2];
end
if((t>=39.5)&&(t<=40.5))
    Wc=[0;0;pi/2];
end
if((t>=59.5)&&(t<=60.5))
    Wc=[0;0;pi/2];
end
dRcdt=R*Skew(Wc);
end

== matlab function NlinCloopintcontrol/Controller1 ==
  data: Pe input; T output; Ve input; Le input; Wcmd output; K parameter
function [T,Wcmd]=Controller(Pe,Ve,Le,K)
x=[Pe;Ve;Le];
u=-K*x;
T=u(1);
Wcmd=u(2:4);
end

== matlab function NlinCloopintcontrol/Trajectory Generator2/MATLAB Function1 ==
  data: R input; dPdt output; t input; Vc output
function [dPdt,Vc] = dPdt(R,t)
Vc=[0.5;0;0];
dPdt=R*Vc;
end

== matlab function NlinCloopintcontrol/Controller3/Controller ==
  data: Pe input; T output; Ve input; Le input; Wcmd output; Ki parameter; Yi input; dYidt output; x output; u output
function [T,Wcmd,dYidt,x,u]=Controller(Pe,Ve,Le,Ki,Yi)
x=[Pe;Ve;Le;Yi];
u=-Ki*x;
T=u(1);
Wcmd=u(2:4);
dYidt=[Pe;Le(3)];
end

== matlab function NlinCloopintcontrol/NTL3 ==
  data: Vc input; Pe output; Wc input; Rc input; Pc input; V input; W input; R input; P input; Ve output; Le output; Lc output; L output
function [Pe,Ve,Le,Lc,L] = NLT(Vc,Wc,Rc,Pc,V,W,R,P)
Rc2b=R'*Rc;
Ve=V-Vc;
Re=Rc'*R;
%Pe=R'*(P-Pc);
Pe=R'*(P-Pc);
L=Rmat2PRY(R)*180/pi;
Lc=Rmat2PRY(Rc)*180/pi;
Le=Rmat2PRY(Re);
end

== matlab function NlinCloopintcontrol/Quadrotor3/MATLAB Function ==
  data: Wcmd input; N output; W input
function N = Wcontorl(Wcmd,W)
N=1000*(Wcmd-W);
end

== matlab function NlinCloopintcontrol/Quadrotor3/MATLAB Function1 ==
  data: V input; dVdt output; W input; R input; T input; N input; dWdt output; Jinv parameter; m parameter; g parameter; J parameter; windforce parameter
function [dVdt,dWdt]=QDyanamics(V,W,R,T,N,Jinv, m, g, J, windforce)
dVdt=-Skew(W)*V+1/m*([0;0;-T]+R'*[0;0;m*g]+ windforce);
dWdt=-Jinv*Skew(W)*J*W+Jinv*N;
end

== matlab function NlinCloopintcontrol/Quadrotor3/MATLAB Function2 ==
  data: R input; dRdt output; W input
function dRdt=dRdt(R,W)
dRdt=R*Skew(W);
end

== matlab function NlinCloopintcontrol/Quadrotor3/MATLAB Function3 ==
  data: R input; dPdt output; V input
function dPdt=dPdt(R,V)
dPdt=R*V;
end

== matlab function NlinCloopintcontrol/Trajectory Generator3/MATLAB Function ==
  data: R input; dRcdt output; t input; Wc output
function [dRcdt,Wc] =dRdt(R,t)

Wc=[0;0;0];
if((t>=19.5)&&(t<=20.5))
    Wc=[0;0;pi/2];
end
if((t>=39.5)&&(t<=40.5))
    Wc=[0;0;pi/2];
end
if((t>=59.5)&&(t<=60.5))
    Wc=[0;0;pi/2];
end
dRcdt=R*Skew(Wc);
end

== matlab function NlinCloopintcontrol/Trajectory Generator3/MATLAB Function1 ==
  data: R input; dPdt output; t input; Vc output
function [dPdt,Vc] = dPdt(R,t)
Vc=[0.5;0;0];
dPdt=R*Vc;
end

== matlab function NlinCloopintcontrol/Controller4/Controller ==
  data: Pe input; T output; Ve input; Le input; Wcmd output; Ki parameter; Yi input; dYidt output
function [T,Wcmd,dYidt]=Controller(Pe,Ve,Le,Ki,Yi)
x=[Pe;Ve;Le;Yi];
u=-Ki*x;
T=u(1);
Wcmd=u(2:4);
dYidt=[Pe;Le(3)];
end

== matlab function NlinCloopintcontrol/Trajectory Generator/MATLAB Function1 ==
  data: R input; dPdt output; t input; Vc output
function [dPdt,Vc] = dPdt(R,t)
Vc=[0.5;0;0];
dPdt=R*Vc;
end

== matlab function NlinCloopintcontrol/NTL4 ==
  data: Vc input; Pe output; Wc input; Rc input; Pc input; V input; W input; R input; P input; Ve output; Le output; Lc output; L output
function [Pe,Ve,Le,Lc,L] = NLT(Vc,Wc,Rc,Pc,V,W,R,P)
Rc2b=R'*Rc;
Ve=V-Vc;
Re=Rc'*R;
%Pe=R'*(P-Pc);
Pe=R'*(P-Pc);
L=Rmat2PRY(R)*180/pi;
Lc=Rmat2PRY(Rc)*180/pi;
Le=Rmat2PRY(Re);
end

== matlab function NlinCloopintcontrol/Quadrotor4/MATLAB Function ==
  data: Wcmd input; N output; W input
function N = Wcontorl(Wcmd,W)
N=1000*(Wcmd-W);
end

== matlab function NlinCloopintcontrol/Quadrotor4/MATLAB Function1 ==
  data: V input; dVdt output; W input; R input; T input; N input; dWdt output; Jinv parameter; m parameter; g parameter; J parameter; windforce parameter
function [dVdt,dWdt]=QDyanamics(V,W,R,T,N,Jinv, m, g, J, windforce)
dVdt=-Skew(W)*V+1/m*([0;0;-T]+R'*[0;0;m*g]+windforce);
dWdt=-Jinv*Skew(W)*J*W+Jinv*N;
end

== matlab function NlinCloopintcontrol/Quadrotor4/MATLAB Function2 ==
  data: R input; dRdt output; W input
function dRdt=dRdt(R,W)
dRdt=R*Skew(W);
end

== matlab function NlinCloopintcontrol/Quadrotor4/MATLAB Function3 ==
  data: R input; dPdt output; V input
function dPdt=dPdt(R,V)
dPdt=R*V;
end

== matlab function NlinCloopintcontrol/Trajectory Generator4/MATLAB Function ==
  data: R input; dRcdt output; t input; Wc output
function [dRcdt,Wc] =dRdt(R,t)

Wc=[0;0;0];
if((t>=19.5)&&(t<=20.5))
    Wc=[0;0;pi/2];
end
if((t>=39.5)&&(t<=40.5))
    Wc=[0;0;pi/2];
end
if((t>=59.5)&&(t<=60.5))
    Wc=[0;0;pi/2];
end
dRcdt=R*Skew(Wc);
end

== matlab function NlinCloopintcontrol/Trajectory Generator4/MATLAB Function1 ==
  data: R input; dPdt output; t input; Vc output
function [dPdt,Vc] = dPdt(R,t)
Vc=[0.5;0;0];
dPdt=R*Vc;
end

== matlab function NlinCloopintcontrol/Controller /Controller ==
  data: Pe input; T output; Ve input; Le input; Wcmd output; Ki parameter; Yi input; dYidt output
function [T,Wcmd,dYidt]=Controller(Pe,Ve,Le,Ki,Yi)
x=[Pe;Ve;Le;Yi];
u=-Ki*x;
T=u(1);
Wcmd=u(2:4);
dYidt=[Pe;Le(3)];
end

== matlab function NlinCloopintcontrol/Quadrotor/MATLAB Function ==
  data: Wcmd input; N output; W input
function N = Wcontorl(Wcmd,W)
N=1000*(Wcmd-W);
end

== matlab function NlinCloopintcontrol/NTL  ==
  data: Rc input; Vc input; Pe output; Wc input; Pc input; P input; V input; R input; W input; Ve output; Le output; Lc output; L output
function [Pe,Ve,Le,Lc,L] = NLT(Rc,Vc,Wc,Pc,P,V,R,W)
Rc2b=R'*Rc;
Ve=V-Vc;
Re=Rc'*R;
%Pe=R'*(P-Pc);
Pe=R'*(P-Pc);
L=Rmat2PRY(R)*180/pi;
Lc=Rmat2PRY(Rc)*180/pi;
Le=Rmat2PRY(Re);
end

== matlab function NlinCloopintcontrol/Quadrotor /MATLAB Function ==
  data: Wcmd input; N output; W input
function N = Wcontorl(Wcmd,W)
N=1000*(Wcmd-W);
end

== matlab function NlinCloopintcontrol/Quadrotor /MATLAB Function1 ==
  data: V input; dVdt output; W input; R input; T input; N input; dWdt output; Jinv parameter; m parameter; g parameter; J parameter; windforce parameter
function [dVdt,dWdt]=QDyanamics(V,W,R,T,N,Jinv, m, g, J, windforce)
dVdt=-Skew(W)*V+1/m*([0;0;-T]+R'*[0;0;m*g]+windforce);
dWdt=-Jinv*Skew(W)*J*W+Jinv*N;
end

== matlab function NlinCloopintcontrol/Quadrotor /MATLAB Function2 ==
  data: R input; dRdt output; W input
function dRdt=dRdt(R,W)
dRdt=R*Skew(W);
end

== matlab function NlinCloopintcontrol/Quadrotor /MATLAB Function3 ==
  data: R input; dPdt output; V input
function dPdt=dPdt(R,V)
dPdt=R*V;
end

== matlab function NlinCloopintcontrol/Trajectory Generator /MATLAB Function ==
  data: R input; dRcdt output; t input; Wc output
function [dRcdt,Wc] =dRdt(R,t)

Wc=[0;0;0];
if((t>=19.5)&&(t<=20.5))
    Wc=[0;0;pi/2];
end
if((t>=39.5)&&(t<=40.5))
    Wc=[0;0;pi/2];
end
if((t>=59.5)&&(t<=60.5))
    Wc=[0;0;pi/2];
end
dRcdt=R*Skew(Wc);
end

== matlab function NlinCloopintcontrol/Trajectory Generator /MATLAB Function1 ==
  data: R input; dPdt output; t input; Vc output
function [dPdt,Vc] = dPdt(R,t)
Vc=[0.5;0;0];
dPdt=R*Vc;
end

== matlab function NlinCloopintcontrol/Quadrotor/MATLAB Function1 ==
  data: V input; dVdt output; W input; R input; T input; N input; dWdt output; Jinv parameter; m parameter; g parameter; J parameter; windforce parameter
function [dVdt,dWdt]=QDyanamics(V,W,R,T,N,Jinv, m, g, J, windforce)
dVdt=-Skew(W)*V+1/m*([0;0;-T]+R'*[0;0;m*g]+windforce);
dWdt=-Jinv*Skew(W)*J*W+Jinv*N;
end

== matlab function NlinCloopintcontrol/Quadrotor/MATLAB Function2 ==
  data: R input; dRdt output; W input
function dRdt=dRdt(R,W)
dRdt=R*Skew(W);
end

== matlab function NlinCloopintcontrol/Quadrotor/MATLAB Function3 ==
  data: R input; dPdt output; V input
function dPdt=dPdt(R,V)
dPdt=R*V;
end

== matlab function NlinCloopintcontrol/NTL ==
  data: Vc input; Pe output; Wc input; Rc input; Pc input; V input; W input; R input; P input; Ve output; Le output; Lc output; L output
function [Pe,Ve,Le,Lc,L] = NLT(Vc,Wc,Rc,Pc,V,W,R,P)
Rc2b=R'*Rc;
Ve=V-Vc;
Re=Rc'*R;
%Pe=R'*(P-Pc);
Pe=R'*(P-Pc);
L=Rmat2PRY(R)*180/pi;
Lc=Rmat2PRY(Rc)*180/pi;
Le=Rmat2PRY(Re);
end
